simulink subsystem "Sensors"  (R2023b)
settings: Solver=VariableStepAuto  StartTime=0.0  StopTime=10.0  RelTol=1e-3
undefined symbols (not defined in the file): Ts
libraries: nesl_utility x2, mcbhdlpositiondecoderlib x1
settings Model: DataDictionary=data_interface.sldd  EnableAccessToBaseWorkspace=off  Creator=upattacini  LastModifiedBy=upattacini

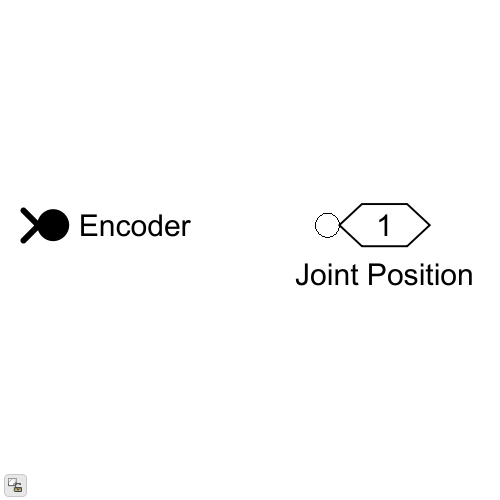
[thumbnail: Simulink's stored preview of the top-level diagram]
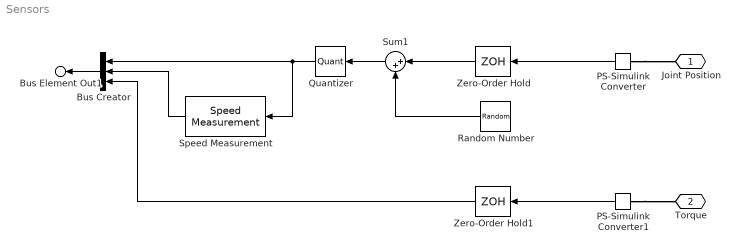
== system Sensors ==
  Bus Creator : BusCreator  Inputs=3  OutDataTypeStr=Bus: Joint_Feedback  NonVirtualBus=on
      settings: InheritFromInputs=off
  PS-Simulink Converter : nesl_utility/PS-Simulink Converter  PhysicalDomain=network_engine_domain  SubClassName=ps_output  LeftPortType=input  RightPortType=output  PseudoPeriodic=off  Frequencies=[]  VectorFormat=inherit  Unit=deg  AffineConversion=off
  PS-Simulink Converter1 : nesl_utility/PS-Simulink Converter  PhysicalDomain=network_engine_domain  SubClassName=ps_output  LeftPortType=input  RightPortType=output  PseudoPeriodic=off  Frequencies=[]  VectorFormat=inherit  Unit=N*m  AffineConversion=off
  Quantizer : Quantizer  QuantizationInterval=360/(2^14)
  Random Number : RandomNumber  Variance=3e-4  SampleTime=Ts
  Speed Measurement : mcbhdlpositiondecoderlib/Speed Measurement  PositionUnit=Degrees  PositionScalingDatatype=uint32  SpeedCalculationMode=Time interval for speed calculation  SampleTimeAsync=Ts  MaximumApplicationSpeed=1000  SpeedResolution=5e-6  DelayLength=40  MaximumMeasurableSpeed=749  MeasurableSpeedResolution=3.4925e-07  SpeedUnit=Degrees/Sec  PerUnitSpeed=1000  SpeedDataType=double
      settings: LibrarySourceBlock=mcbhdllib/Sensor Decoders/Speed Measurement
  Sum1 : Sum  Inputs=|++
  Zero-Order Hold : ZeroOrderHold  SampleTime=Ts
  Zero-Order Hold1 : ZeroOrderHold  SampleTime=Ts
  Joint Position : PMIOPort  Side=Right
  Torque : PMIOPort  Port=2  Side=Right
  Bus Element Out1 : Outport  PortName=Joint Feedback
  wires:
  Zero-Order Hold/1 -> Sum1/1
  Sum1/1 -> Quantizer/1
  Random Number/1 -> Sum1/2
  Quantizer/1 -> Bus Creator/1, Speed Measurement/1
  PS-Simulink Converter/1 -> Zero-Order Hold/1
  Bus Creator/1 -> Bus Element Out1/1
  Speed Measurement/1 -> Bus Creator/2
  PS-Simulink Converter1/1 -> Zero-Order Hold1/1
  Zero-Order Hold1/1 -> Bus Creator/3
  connections:
  PS-Simulink Converter/LConn1 -- Joint Position/RConn1
  PS-Simulink Converter1/LConn1 -- Torque/RConn1
